simulink model "State_Flow_TestM"  (R2017a)
settings: Solver=FixedStepDiscrete  StartTime=0.0  StopTime=inf  FixedStep=0.001  RelTol=1e-3  EnableMultiTasking=on
values from neighbouring files (symbols this model uses):
  C = B    [testMatricePiccola.m]
libraries: xpcethercatlib x33, simulink x17, powerlib_meascontrol x3, commutil2 x2
(part 2 of 4)

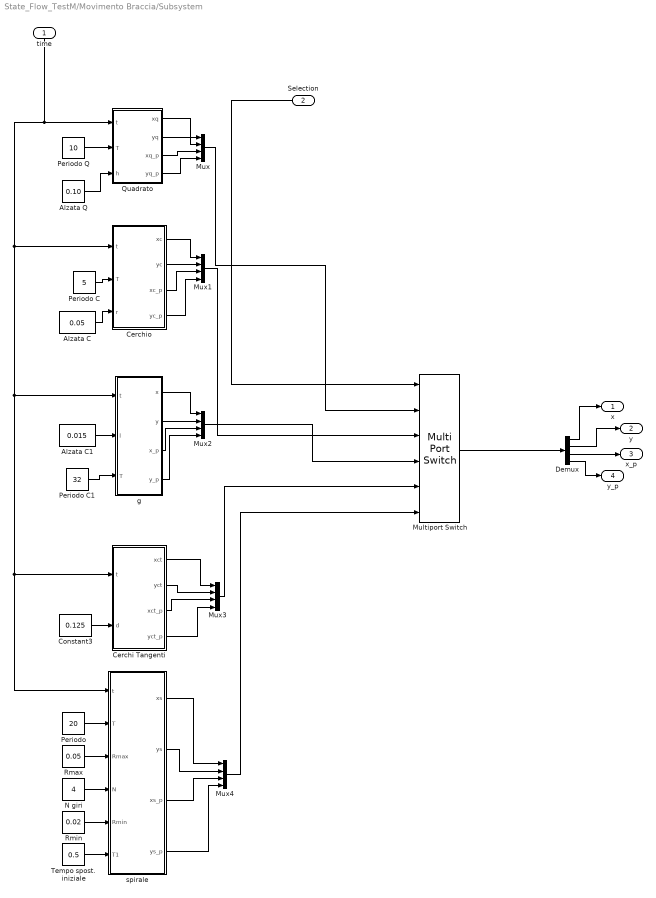
== system State_Flow_TestM/Movimento Braccia/Subsystem ==
  time : Inport
  Selection : Inport  Port=2
  Alzata C : Constant  Value=0.05
  Alzata C1 : Constant  Value=0.015
  Alzata Q : Constant  Value=0.10
  Cerchi Tangenti : MATLAB Function  TreatAsAtomicUnit=on
  Cerchio : MATLAB Function  TreatAsAtomicUnit=on
  Constant3 : Constant  Value=0.125
  Demux : Demux
  Multiport Switch : MultiPortSwitch  Inputs=5
  Mux{,1..4} (5 alike) : Mux
  N giri : Constant  Value=4
  Periodo : Constant  Value=20
  Periodo C : Constant  Value=5
  Periodo C1 : Constant  Value=32
  Periodo Q : Constant  Value=10
  Quadrato : MATLAB Function  TreatAsAtomicUnit=on
  Rmax : Constant  Value=0.05
  Rmin : Constant  Value=0.02
  Tempo spost. iniziale : Constant  Value=0.5
  g : MATLAB Function  TreatAsAtomicUnit=on
  spirale : MATLAB Function  TreatAsAtomicUnit=on
  x : Outport
  y : Outport  Port=2
  x_p : Outport  Port=3
  y_p : Outport  Port=4
  wires:
  Cerchio/2(yc) -> Mux1/2
  Cerchio/3(xc_p) -> Mux1/3
  Cerchio/4(yc_p) -> Mux1/4
  Cerchio/1(xc) -> Mux1/1
  Mux4/1 -> Multiport Switch/6
  Mux2/1 -> Multiport Switch/4
  spirale/4(ys_p) -> Mux4/4
  Quadrato/2(yq) -> Mux/2
  Quadrato/3(xq_p) -> Mux/3
  Quadrato/4(yq_p) -> Mux/4
  g/1(x) -> Mux2/1
  Demux/2 -> y/1
  Demux/1 -> x/1
  Selection/1 -> Multiport Switch/1
  time/1 -> Quadrato/1(t), Cerchio/1(t), g/1(t), Cerchi Tangenti/1(t), spirale/1(t)
  spirale/3(xs_p) -> Mux4/3
  spirale/2(ys) -> Mux4/2
  g/3(x_p) -> Mux2/3
  g/4(y_p) -> Mux2/4
  Cerchi Tangenti/2(yct) -> Mux3/2
  Cerchi Tangenti/1(xct) -> Mux3/1
  Cerchi Tangenti/4(yct_p) -> Mux3/4
  Cerchi Tangenti/3(xct_p) -> Mux3/3
  Quadrato/1(xq) -> Mux/1
  g/2(y) -> Mux2/2
  spirale/1(xs) -> Mux4/1
  Periodo C/1 -> Cerchio/2(T)
  Periodo Q/1 -> Quadrato/2(T)
  Alzata C/1 -> Cerchio/3(r)
  Alzata Q/1 -> Quadrato/3(h)
  Periodo/1 -> spirale/2(T)
  Constant3/1 -> Cerchi Tangenti/2(d)
  N giri/1 -> spirale/4(N)
  Rmin/1 -> spirale/5(Rmin)
  Tempo spost. iniziale/1 -> spirale/6(T1)
  Alzata C1/1 -> g/2(l)
  Periodo C1/1 -> g/3(T)
  Rmax/1 -> spirale/3(Rmax)
  Multiport Switch/1 -> Demux/1
  Mux3/1 -> Multiport Switch/5
  Mux/1 -> Multiport Switch/2
  Mux1/1 -> Multiport Switch/3
  Demux/3 -> x_p/1
  Demux/4 -> y_p/1

== system State_Flow_TestM/Movimento Braccia/Velocita vite  ==
  EtherCAT PDO Receive14 : xpcethercatlib/EtherCAT PDO Receive  Priority=2  sig_name=AZ1.Transmit PDO 1.Axis A Actual motor velocity  sig_offset=48  sig_type=int32  type_size=32  sig_dim=1  device_id=0  sample_time=0.001000
      settings: SourceProductName=Simulink Real-Time  SourceProductBaseCode=XP
  EtherCAT PDO Receive15 : xpcethercatlib/EtherCAT PDO Receive  Priority=2  sig_name=AZ1.Transmit PDO 2.Axis B Actual motor velocity  sig_offset=136  sig_type=int32  type_size=32  sig_dim=1  device_id=0  sample_time=0.001000
      settings: SourceProductName=Simulink Real-Time  SourceProductBaseCode=XP
  Vel Asse A conv : MATLAB Function  TreatAsAtomicUnit=on
  Vel Asse B conv : MATLAB Function  TreatAsAtomicUnit=on
  Velocity A : DataTypeConversion
  Velocity B : DataTypeConversion
  Asse B : Outport
  Asse A : Outport  Port=2
  wires:
  EtherCAT PDO Receive15/1 -> Velocity B/1
  EtherCAT PDO Receive14/1 -> Velocity A/1
  Vel Asse A conv/1(vel_A_conv) -> Asse A/1
  Velocity B/1 -> Vel Asse B conv/1(p)
  Vel Asse B conv/1(vel_B_conv) -> Asse B/1
  Velocity A/1 -> Vel Asse A conv/1(vA)

== system State_Flow_TestM/Out Asse A Braccia/Fungo ==
  In1 : Inport
  Constant : Constant  Value=0
  Data Type Conversion14 : DataTypeConversion
  Display10 : Display
  EtherCAT PDO Receive9 : xpcethercatlib/EtherCAT PDO Receive  Priority=2  sig_name=Beckoff.Channel 1.Input  sig_offset=0  sig_type=boolean  type_size=1  sig_dim=1  device_id=0  sample_time=0.001000
      settings: SourceProductName=Simulink Real-Time  SourceProductBaseCode=XP
  MATLAB Function : MATLAB Function  TreatAsAtomicUnit=on
  Memory : Memory
  Switch1 : Switch  Criteria=u2 ~= 0  Threshold=2
  Out1 : Outport
  wires:
  EtherCAT PDO Receive9/1 -> Data Type Conversion14/1
  Data Type Conversion14/1 -> MATLAB Function/2(old), Display10/1
  MATLAB Function/1(y) -> Memory/1
  In1/1 -> Switch1/3
  Memory/1 -> Switch1/2, MATLAB Function/1(now)
  Constant/1 -> Switch1/1
  Switch1/1 -> Out1/1

== system State_Flow_TestM/Out Asse B Braccia/Fungo ==
  In1 : Inport
  Constant : Constant  Value=0
  Data Type Conversion14 : DataTypeConversion
  Display10 : Display
  EtherCAT PDO Receive9 : xpcethercatlib/EtherCAT PDO Receive  Priority=2  sig_name=Beckoff.Channel 1.Input  sig_offset=0  sig_type=boolean  type_size=1  sig_dim=1  device_id=0  sample_time=0.001000
      settings: SourceProductName=Simulink Real-Time  SourceProductBaseCode=XP
  MATLAB Function : MATLAB Function  TreatAsAtomicUnit=on
  Memory : Memory
  Switch1 : Switch  Criteria=u2 ~= 0  Threshold=2
  Out1 : Outport
  wires:
  EtherCAT PDO Receive9/1 -> Data Type Conversion14/1
  Data Type Conversion14/1 -> MATLAB Function/2(old), Display10/1
  MATLAB Function/1(y) -> Memory/1
  In1/1 -> Switch1/3
  Memory/1 -> Switch1/2, MATLAB Function/1(now)
  Constant/1 -> Switch1/1
  Switch1/1 -> Out1/1

== system State_Flow_TestM/Out asse A Vite/Fungo ==
  In1 : Inport
  Constant : Constant  Value=0
  Data Type Conversion14 : DataTypeConversion
  Display10 : Display
  EtherCAT PDO Receive9 : xpcethercatlib/EtherCAT PDO Receive  Priority=2  sig_name=Beckoff.Channel 1.Input  sig_offset=0  sig_type=boolean  type_size=1  sig_dim=1  device_id=0  sample_time=0.001000
      settings: SourceProductName=Simulink Real-Time  SourceProductBaseCode=XP
  MATLAB Function : MATLAB Function  TreatAsAtomicUnit=on
  Memory : Memory
  Switch1 : Switch  Criteria=u2 ~= 0  Threshold=2
  Out1 : Outport
  wires:
  EtherCAT PDO Receive9/1 -> Data Type Conversion14/1
  Data Type Conversion14/1 -> MATLAB Function/2(old), Display10/1
  MATLAB Function/1(y) -> Memory/1
  In1/1 -> Switch1/3
  Memory/1 -> Switch1/2, MATLAB Function/1(now)
  Constant/1 -> Switch1/1
  Switch1/1 -> Out1/1

== system State_Flow_TestM/Out asse B Vite/Fungo ==
  In1 : Inport
  Constant : Constant  Value=0
  Data Type Conversion14 : DataTypeConversion
  Display10 : Display
  EtherCAT PDO Receive9 : xpcethercatlib/EtherCAT PDO Receive  Priority=2  sig_name=Beckoff.Channel 1.Input  sig_offset=0  sig_type=boolean  type_size=1  sig_dim=1  device_id=0  sample_time=0.001000
      settings: SourceProductName=Simulink Real-Time  SourceProductBaseCode=XP
  MATLAB Function : MATLAB Function  TreatAsAtomicUnit=on
  Memory : Memory
  Switch1 : Switch  Criteria=u2 ~= 0  Threshold=2
  Out1 : Outport
  wires:
  EtherCAT PDO Receive9/1 -> Data Type Conversion14/1
  Data Type Conversion14/1 -> MATLAB Function/2(old), Display10/1
  MATLAB Function/1(y) -> Memory/1
  In1/1 -> Switch1/3
  Memory/1 -> Switch1/2, MATLAB Function/1(now)
  Constant/1 -> Switch1/1
  Switch1/1 -> Out1/1

== system State_Flow_TestM/Sistema Braccia Linea/Velocita vite  ==
  EtherCAT PDO Receive14 : xpcethercatlib/EtherCAT PDO Receive  Priority=2  sig_name=AZ1.Transmit PDO 1.Axis A Actual motor velocity  sig_offset=48  sig_type=int32  type_size=32  sig_dim=1  device_id=0  sample_time=0.001000
      settings: SourceProductName=Simulink Real-Time  SourceProductBaseCode=XP
  EtherCAT PDO Receive15 : xpcethercatlib/EtherCAT PDO Receive  Priority=2  sig_name=AZ1.Transmit PDO 2.Axis B Actual motor velocity  sig_offset=136  sig_type=int32  type_size=32  sig_dim=1  device_id=0  sample_time=0.001000
      settings: SourceProductName=Simulink Real-Time  SourceProductBaseCode=XP
  Vel Asse A conv : MATLAB Function  TreatAsAtomicUnit=on
  Vel Asse B conv : MATLAB Function  TreatAsAtomicUnit=on
  Velocity A : DataTypeConversion
  Velocity B : DataTypeConversion
  Asse A : Outport
  Asse B : Outport  Port=2
  wires:
  EtherCAT PDO Receive15/1 -> Velocity B/1
  EtherCAT PDO Receive14/1 -> Velocity A/1
  Vel Asse A conv/1(vel_A_conv) -> Asse A/1
  Velocity B/1 -> Vel Asse B conv/1(p)
  Vel Asse B conv/1(vel_B_conv) -> Asse B/1
  Velocity A/1 -> Vel Asse A conv/1(vA)

== system State_Flow_TestM/Sistema Vite/Actual A ==
  Pos : Inport
  Offset : Inport  Port=2
  Rif asse B : Inport  Port=3
  Discrete Derivative A : simulink/Discrete/Discrete Derivative  gainval=1.0  ICPrevScaledInput=0.0  OutMin=[]  OutMax=[]  OutDataType=fixdt(1, 16)  OutScaling=2^-10  DoSatur=off
  Display31 : Display
  Posizione attuale Vite A : Subsystem
  Sum : Sum  Inputs=|-+
  A attuale : Outport
  wires:
  Offset/1 -> Sum/1
  Posizione attuale Vite A/1(A Att) -> A attuale/1, Discrete Derivative A/1
  Sum/1 -> Posizione attuale Vite A/1(Comp Vite A)
  Rif asse B/1 -> Posizione attuale Vite A/2("Comp Vite B ")
  Pos/1 -> Sum/2
  Discrete Derivative A/1 -> Display31/1

== system State_Flow_TestM/Sistema Vite/Clock reale ==
  cr : Inport
  offset : Inport  Port=2
  Sum2 : Sum  Inputs=-+|
  Ck : Outport
  wires:
  Sum2/1 -> Ck/1
  offset/1 -> Sum2/1
  cr/1 -> Sum2/2

== system State_Flow_TestM/Sistema Vite/Coppia VIte A finale ==
  Pos : Inport
  Vel : Inport  Port=2
  Gain : Gain  Gain=300*1000/0.36
  Gain6 : Gain  Gain=7.5*1000/0.36
  Sum9 : Sum  Inputs=|++
  Coppia : Outport
  wires:
  Pos/1 -> Gain/1
  Sum9/1 -> Coppia/1
  Gain6/1 -> Sum9/2
  Vel/1 -> Gain6/1
  Gain/1 -> Sum9/1

== system State_Flow_TestM/Sistema Vite/Velocita vite  ==
  EtherCAT PDO Receive14 : xpcethercatlib/EtherCAT PDO Receive  Priority=2  sig_name=AZ2.Transmit PDO 1.Axis A Actual motor velocity  sig_offset=304  sig_type=int32  type_size=32  sig_dim=1  device_id=0  sample_time=0.001000
      settings: SourceProductName=Simulink Real-Time  SourceProductBaseCode=XP
  EtherCAT PDO Receive15 : xpcethercatlib/EtherCAT PDO Receive  Priority=2  sig_name=AZ2.Transmit PDO 2.Axis B Actual motor velocity  sig_offset=392  sig_type=int32  type_size=32  sig_dim=1  device_id=0  sample_time=0.001000
      settings: SourceProductName=Simulink Real-Time  SourceProductBaseCode=XP
  Vel Asse A conv : MATLAB Function  TreatAsAtomicUnit=on
  Vel Asse B conv : MATLAB Function  TreatAsAtomicUnit=on
  Velocity A : DataTypeConversion
  Velocity B : DataTypeConversion
  Asse A : Outport
  Asse B : Outport  Port=2
  wires:
  EtherCAT PDO Receive15/1 -> Velocity B/1
  EtherCAT PDO Receive14/1 -> Velocity A/1
  Vel Asse A conv/1(vel_A_conv) -> Asse A/1
  Velocity B/1 -> Vel Asse B conv/1(p), Vel Asse A conv/2(vB)
  Vel Asse B conv/1(vel_B_conv) -> Asse B/1
  Velocity A/1 -> Vel Asse A conv/1(vA)

== system State_Flow_TestM/State flow robot/Mov1/Clock reale ==
  cr : Inport
  offset : Inport  Port=2
  Sum2 : Sum  Inputs=-+|
  Ck : Outport
  wires:
  Sum2/1 -> Ck/1
  offset/1 -> Sum2/1
  cr/1 -> Sum2/2

== system State_Flow_TestM/Sistema Vite/Actual A/Posizione attuale Vite A ==
  Comp Vite A : Inport
  "Comp Vite B " : Inport  Port=2
  Asse A conv : MATLAB Function  TreatAsAtomicUnit=on
  Asse B conv v : MATLAB Function  TreatAsAtomicUnit=on
  Sum5 : Sum
  A Att : Outport
  wires:
  Asse A conv/1(pos_A_conv) -> Sum5/1
  Asse B conv v/1(pos_B_conv_v) -> Sum5/2
  Comp Vite A/1 -> Asse A conv/1(p)
  Sum5/1 -> A Att/1
  "Comp Vite B "/1 -> Asse B conv v/1(p)

== matlab function State_Flow_TestM/Movimento Braccia/Cinematica Inversa1 ==
  data: x0old input; y0old input; theta1_0 input; theta2_0 input; time input; x0 output; y0 output
function [x0, y0] = fcn(x0old, y0old, theta1_0, theta2_0, time)

if time == 0 

d = 0.09; 
l = 0.25;

A = l^2*(sin(theta2_0)-sin(theta1_0))^2 + (-2*d -l*(cos(theta2_0)-cos(theta1_0)))^2;
B = -2*l^2*d*(sin(theta2_0)-sin(theta1_0))*(cos(theta2_0)+cos(theta1_0)) + ...
    l*(sin(theta2_0)-sin(theta1_0))*(-2*d -l*(cos(theta2_0)-cos(theta1_0)))*(-2*d -2*l*cos(theta2_0)) - ...
    2*l*sin(theta2_0)*(-2*d -l*(cos(theta2_0)-cos(theta1_0)))^2;
C = l^2*d^2*(cos(theta2_0)+cos(theta1_0))^2 -l*d*(cos(theta2_0)+cos(theta1_0))*(-2*d -l*(cos(theta2_0)-cos(theta1_0)))*(-2*d -2*l*cos(theta2_0)) + ...
    (d^2 + 2*d*l*cos(theta2_0))*(-2*d - l*(cos(theta2_0)-cos(theta1_0)))^2;

% Posizione Y end-effector
y0 = (-B + sqrt(B^2 - 4*A*C))/(2*A);
% Posizione X end-effector
x0 = (y0*l*(sin(theta2_0)-sin(theta1_0)) - l*d*(cos(theta2_0)+cos(theta1_0)))/(-2*d -l*(cos(theta2_0)-cos(theta1_0)));
else 
    x0 = x0old;
    y0 = y0old;
end

== matlab function State_Flow_TestM/Movimento Braccia/MATLAB Function ==
  data: x input; xp output; y input; yp output; bool input
function [xp,yp] = fcn(x, y, bool)
if bool == 4
    xp = x;
    yp = y;
else
    xp = 0;
    yp = 0;
end

== matlab function State_Flow_TestM/Sistema Braccia Linea/Velocita vite /Vel Asse A conv ==
  data: vA input; vel_A_conv output
function vel_A_conv = fcn(vA)
vel_A_conv = (vA)  *(2*pi)/163840/64;

== matlab function State_Flow_TestM/Sistema Braccia Linea/Velocita vite /Vel Asse B conv ==
  data: p input; vel_B_conv output
function vel_B_conv = fcn(p)
vel_B_conv = p  *(2*pi)/163840/64;

== matlab function State_Flow_TestM/Sistema Vite/Actual A/Posizione attuale Vite A/Asse A conv ==
  data: p input; pos_A_conv output
function pos_A_conv = fcn(p)
pos_A_conv = p * 0.02/(2*pi) * pi/2048/40;

== matlab function State_Flow_TestM/Sistema Vite/Rifermento Asse A Vite ==
  data: t input; ldm_pos output; h input; T input; ldm_vel output
function [ldm_pos, ldm_vel] = fcn(t,h,T)

xv = 0.3;
 x = t/T;
Ca=1/(xv*(1-xv));
Cv = 1/(1-xv);

if( x>= 0 && x < xv)
    f = Ca;
    F = Ca*x;
    G= Ca*x^2/2;
elseif(x >= xv && x < (1-xv) )
    f = 0;
    F = Cv;
    G= Ca*xv^2/2 + Cv*(x-xv);
elseif( x >= (1-xv) && x <= 1 )
    f = -Ca;
    xloc = x-(1-xv);
    F = Cv -Ca*xloc;
    G= Ca*xv^2/2 + Cv*(1-2*xv) + Cv*xloc -Ca*xloc^2/2;
else
    f=0;
    F=0;
    G= Ca*xv^2/2 + Cv*(1-2*xv) + Cv*xv -Ca*xv^2/2;
end

ldm_pos = G*h;
ldm_vel = F*h/T;

== matlab function State_Flow_TestM/LED Status/MATLAB Function ==
  data: u input; y output
function y = fcn(u)
if u == 2 ||u == 3
    y = 1;
else
    y = 0;
end

== matlab function State_Flow_TestM/LED Status/MATLAB Function1 ==
  data: u input; y output
function y = fcn(u)
if u == 1 || u == 2 || u == 4
    y = 1;
else
    y = 0;
end

== matlab function State_Flow_TestM/LED Status/MATLAB Function2 ==
  data: u input; y output
function y = fcn(u)
if u == 4 || u == 5
    y = 1;
else
    y = 0;
end

== matlab function State_Flow_TestM/Sistema Vite/Asse B conv ==
  data: p input; pos_B_conv output
function pos_B_conv = fcn(p)
pos_B_conv = p * pi/2048/40;

== matlab function State_Flow_TestM/Sistema Vite/Asse B ==
  data: t input; ldm_pos output; h input; T input; ldm_vel output
function [ldm_pos, ldm_vel] = fcn(t,h,T)

xv = 0.3;
 x = t/T;
Ca=1/(xv*(1-xv));
Cv = 1/(1-xv);

if( x>= 0 && x < xv)
    f = Ca;
    F = Ca*x;
    G= Ca*x^2/2;
elseif(x >= xv && x < (1-xv) )
    f = 0;
    F = Cv;
    G= Ca*xv^2/2 + Cv*(x-xv);
elseif( x >= (1-xv) && x <= 1 )
    f = -Ca;
    xloc = x-(1-xv);
    F = Cv -Ca*xloc;
    G= Ca*xv^2/2 + Cv*(1-2*xv) + Cv*xloc -Ca*xloc^2/2;
else
    f=0;
    F=0;
    G= Ca*xv^2/2 + Cv*(1-2*xv) + Cv*xv -Ca*xv^2/2;
end

ldm_pos = G*h;
ldm_vel = F*h/T;

== matlab function State_Flow_TestM/Sistema Vite/Actual A/Posizione attuale Vite A/Asse B conv v ==
  data: p input; pos_B_conv_v output
function pos_B_conv_v = fcn(p)
pos_B_conv_v = p * 0.02/(2*pi) * pi/2048/40;

== matlab function State_Flow_TestM/Sistema Vite/Velocita vite /Vel Asse A conv ==
  data: vA input; vel_A_conv output; vB input
function vel_A_conv = fcn(vA, vB)
vel_A_conv = (vA+vB) * 0.02/(2*pi) * pi/20480/40;

== matlab function State_Flow_TestM/Sistema Vite/Velocita vite /Vel Asse B conv ==
  data: p input; vel_B_conv output
function vel_B_conv = fcn(p)
vel_B_conv = p  * pi/20480/40;

== stateflow chart State_Flow_TestM/State flow robot ==
  settings: sampleTime=0.001
  state Step1
    entry:
    Bool = -1;
  state Step2
    entry:
    CoppiaH = 0;
  state SetA
    entry:
    CoppiaA = 0;
    C1 = 0;
  state OffSet
    entry:
    CoppiaH = 0;
    CoppiaA = 0;
    CoppiaB = 0;
    OffA = posA;
    OffB = posB;
    OffA_0 = posA;
    OffB_0 = posB;
    Bool = 2;
    Luci = 3;
    Hv = 1;
  state SetB1
    entry:
    CoppiaB = 0;
    C2 = 0;
  state Discesa_Vite
    entry:
    OffA_vite = posA_vite;
    CoppiaH=700;
  state Traiettoria
    entry:
    OffT = Clock;
    OffA_vite = posA_vite;
    OffB_vite = posB_vite;
    Luci = 4;
    Bool = 4;
    Hb = 1;
  state Step4
    entry:
    Bool = 0;
    Enable = 1;
  state Test_Kp
    entry:
    Bool = 5;
    Luci = 5;
    Kp = Kp + 500;
  state Controllo
    entry:
    Bool = 5;
    Luci = 5;
  state Coppie
    entry:
    OffA_0 = posA;
    OffB_0 = posB;
    CoppiaA = 250;
    CoppiaB = 250;
    CoppiaH = 0;
    Luci = 2;
  state SetB
    entry:
    CoppiaB = 0;
    C2 = 0;
  state SetA1
    entry:
    CoppiaA = 0;
    C1 = 0;
  state Home
    entry:
    [CoppiaA, CoppiaB, CoppiaH] = Homing(fc, fcA, fcB);
    Bool = 1;
    conv =  (2*pi)/16384/64;
    conv_vite = 0.02/(2*pi) * pi/2048/40;
    Luci = 1;
    C1 = 1;
    C2 = 1;
    Kp = KP;
    Hb = 0;
    Hv = 0;
  state Step3
    entry:
    CoppiaA = 0;
    CoppiaB = 0;
  state [CA,CB,CH] = Homing(fc,fcA,fcB) [function]
  state [CA,CB] = Mov1(posA,OffA,posB,OffB,OffT,Clock) [function] [commented out]
  state [CA,CB] = Mov(posA,OffA,posB,OffB,Clock, OffT, velA, velB) [function] [commented out]
  (default) -> Step1
  Step1 -> Step4 : [Status==1079 && avvio == 1]
  Home -> Step2 [order 2] : [fc==0]
  Coppie -> SetA [order 1] : [posA - OffA_0 >= 110*pi/180/conv]
  Step2 -> Coppie : [fcA == 1 && fcB==1]
  Discesa_Vite -> OffSet [order 1] : [posA_vite - OffA_vite >= 0.038/conv_vite]
  SetA -> SetB1 : [posB - OffB_0 >= 40*pi/180/conv]
  SetB1 -> Discesa_Vite : [C2 == 0]
  Traiettoria -> Test_Kp : after(6,sec)
  Test_Kp -> Controllo [order 2] : [Kp >= 7000]
  OffSet -> Traiettoria : [BeginWork == 1]
  Step4 -> Home : [HomeSignal == 1]
  Test_Kp -> OffSet [order 1] : [Kp < 7000]
  SetA1 -> Discesa_Vite : [C1 == 0]
  Discesa_Vite -> ? [order 1]
  SetB -> SetA1 : [posA - OffA_0 >= 110*pi/180/conv]
  Coppie -> SetB [order 2] : [posB - OffB_0 >= 40*pi/180/conv]
  Step3 -> Coppie : [fc==0]
  Home -> Step3 [order 1] : [fcA==1 && fcB==1]
  data: fc function_input double size=1; CA function_output; CB function_output; CH function_output; fcA function_input double size=1; fcB function_input double size=1; posA function_input double size=1; CA function_output double size=1; CB function_output double size=1; OffA function_input double size=1; posB function_input double size=1; OffB function_input double size=1; OffT function_input double size=1; Clock function_input double size=1; CA function_output double size=1; CB function_output double size=1; posA function_input double size=1; OffA function_input double size=1; posB function_input double size=1; OffB function_input double size=1; Clock function_input double size=1; OffT function_input double size=1; velA function_input double size=1; velB function_input double size=1; Clock input; posA_vite input; posB_vite input; SampleTime constant double; Status input; fc input; posA input; posB input; Bool output; OffT output; CoppiaH output; OffA_vite output; OffB_vite output; OffA output; OffB output; CoppiaA output; CoppiaB output; fcA input; fcB input; conv local; Luci output; OffA_0 local; OffB_0 local; C1 local; C2 local; conv_vite local; Kp output; KP input; Hv output; Hb output; HomeSignal input; avvio input; BeginWork input; Enable output

== matlab function State_Flow_TestM/Movimento Braccia/Cinematica Inversa ==
  data: x input; theta1 output; y input; theta2 output
function [theta1, theta2] = fcn(x, y)

d = 0.09; 
l = 0.25;

p = 2*d*l + 2*x*l;
e = 2*y*l;
f = x^2 + d^2 + y^2 + 2*x*d;
a = -2*d*l + 2*x*l;
b = +2*y*l;
c = x^2 + d^2 + y^2 - 2*x*d;



   theta1 = 2*atan2(e + sqrt(p^2 + e^2 -f^2), p +f);


   theta2 = 2*atan2(b - sqrt(a^2 + b^2 -c^2), a +c);
   if (theta2) < -deg2rad(200)
       theta2 = theta2 + 2*pi;
   end

== matlab function State_Flow_TestM/Movimento Braccia/Asse B conv brac1 ==
  data: p input; pos_B_conv output
function pos_B_conv = fcn(p)
pos_B_conv = p * (2*pi)/16384/64;

== matlab function State_Flow_TestM/State flow robot/Homing/MATLAB Function ==
  data: fc input; CA output; fcA input; fcB input; CB output; CH output
function [CA, CB, CH] = fcn(fc, fcA, fcB)

CA = -250;
CB = -250;
CH = -600;

if fc < 1
    CH = 0;
end
if fcA == 1
    CA = 0;
end
if fcB == 1
    CB = 0;
end

== matlab function State_Flow_TestM/Out asse A Vite/Fungo/MATLAB Function ==
  data: now input; old input; y output
function y = fcn(now, old)
if old == 0 && now == 1
    y = 1;
else
    y = old;
end

== matlab function State_Flow_TestM/Out asse B Vite/Fungo/MATLAB Function ==
  data: now input; old input; y output
function y = fcn(now, old)
if old == 0 && now == 1
    y = 1;
else
    y = old;
end

== matlab function State_Flow_TestM/Out Asse A Braccia/Fungo/MATLAB Function ==
  data: now input; old input; y output
function y = fcn(now, old)
if old == 0 && now == 1
    y = 1;
else
    y = old;
end

== matlab function State_Flow_TestM/Out Asse B Braccia/Fungo/MATLAB Function ==
  data: now input; old input; y output
function y = fcn(now, old)
if old == 0 && now == 1
    y = 1;
else
    y = old;
end

== matlab function State_Flow_TestM/State flow robot/Mov/Cinematica Inversa ==
  data: x input; theta1 output; y input; theta2 output
function [theta1, theta2] = fcn(x, y)

d = 0.09; 
l = 0.25;

p = 2*d*l + 2*x*l;
e = 2*y*l;
f = x^2 + d^2 + y^2 + 2*x*d;
a = -2*d*l + 2*x*l;
b = +2*y*l;
c = x^2 + d^2 + y^2 - 2*x*d;



   theta1 = 2*atan2(e + sqrt(p^2 + e^2 -f^2), p +f);


   theta2 = 2*atan2(b - sqrt(a^2 + b^2 -c^2), a +c);
   if (theta2) < -deg2rad(200)
       theta2 = theta2 + 2*pi;
   end

== matlab function State_Flow_TestM/State flow robot/Mov/Cinematica Inversa vel ==
  data: theta1 input; theta2 input; x input; y input; xp input; theta1_p output; yp input; theta2_p output
function [theta1_p, theta2_p] = fcn(theta1, theta2,x, y, xp, yp)

d = 0.09; 
l = 0.25;

N21 = -l*sin(theta1)*(x+d-l*cos(theta1)) + l*cos(theta1)*(y-l*sin(theta1));

N22 = -l*cos(theta2)*(y-l*sin(theta2))*(x+d-l*cos(theta1))/(x-d-l*cos(theta2)) + l*sin(theta2)*(x+d-l*cos(theta1));

D2 = y-l*sin(theta1) - (y-l*sin(theta2))*(x+d-l*cos(theta1))/(x-d-l*cos(theta2));

J21 = N21/D2;

J22 = N22/D2;

J11 = -(y-l*sin(theta2))/(x-d-l*cos(theta2))*(J21);

J12 = -(y-l*sin(theta2))/(x-d-l*cos(theta2))*(J22) -l*sin(theta2) + (y-l*sin(theta2))/(x-d-l*cos(theta2))*(l*cos(theta2));

J = [J11 J12; J21 J22];

theta_p = J^-1 * [xp; yp];
theta1_p = theta_p(1);
theta2_p = theta_p(2);

== matlab function State_Flow_TestM/State flow robot/Mov1/Asse A conv bracc ==
  data: p input; pos_A_conv output
function pos_A_conv = fcn(p)
pos_A_conv = p * (2*pi)/16384/64;

== matlab function State_Flow_TestM/State flow robot/Mov1/Asse A conv bracc1 ==
  data: p input; pos_A_conv output
function pos_A_conv = fcn(p)
pos_A_conv = p * (2*pi)/16384/64;

== matlab function State_Flow_TestM/State flow robot/Mov1/Ldm theta1 ==
  data: t input; theta1 output; T1 input
function theta1 = fcn(t,T1)
theta1 = T1(t*1000);
end

== matlab function State_Flow_TestM/State flow robot/Mov1/Ldm theta2 ==
  data: t input; theta1 output; T1 input
function theta1 = fcn(t,T1)
theta1 = T1(t*1000);
end

== matlab function State_Flow_TestM/State flow robot/Mov/x ==
  data: t input; ldm_pos output; h input; T input; ldm_vel output
function [ldm_pos, ldm_vel] = fcn(t,h,T)

xv = 0.3;
 x = t/T;
Ca=1/(xv*(1-xv));
Cv = 1/(1-xv);

if( x>= 0 && x < xv)
    f = Ca;
    F = Ca*x;
    G= Ca*x^2/2;
elseif(x >= xv && x < (1-xv) )
    f = 0;
    F = Cv;
    G= Ca*xv^2/2 + Cv*(x-xv);
elseif( x >= (1-xv) && x <= 1 )
    f = -Ca;
    xloc = x-(1-xv);
    F = Cv -Ca*xloc;
    G= Ca*xv^2/2 + Cv*(1-2*xv) + Cv*xloc -Ca*xloc^2/2;
else
    f=0;
    F=0;
    G= Ca*xv^2/2 + Cv*(1-2*xv) + Cv*xv -Ca*xv^2/2;
end

ldm_pos = G*h;
ldm_vel = F*h/T;

== matlab function State_Flow_TestM/State flow robot/Mov/Asse A conv bracc2 ==
  data: p input; pos_A_conv output
function pos_A_conv = fcn(p)
pos_A_conv = p * (2*pi)/16384/64;

== matlab function State_Flow_TestM/State flow robot/Mov/y ==
  data: t input; ldm_pos output; h input; T input; ldm_vel output
function [ldm_pos, ldm_vel] = fcn(t,h,T)

xv = 0.3;
 x = t/T;
Ca=1/(xv*(1-xv));
Cv = 1/(1-xv);

if( x>= 0 && x < xv)
    f = Ca;
    F = Ca*x;
    G= Ca*x^2/2;
elseif(x >= xv && x < (1-xv) )
    f = 0;
    F = Cv;
    G= Ca*xv^2/2 + Cv*(x-xv);
elseif( x >= (1-xv) && x <= 1 )
    f = -Ca;
    xloc = x-(1-xv);
    F = Cv -Ca*xloc;
    G= Ca*xv^2/2 + Cv*(1-2*xv) + Cv*xloc -Ca*xloc^2/2;
else
    f=0;
    F=0;
    G= Ca*xv^2/2 + Cv*(1-2*xv) + Cv*xv -Ca*xv^2/2;
end

ldm_pos = G*h;
ldm_vel = F*h/T;

== matlab function State_Flow_TestM/State flow robot/Mov/Asse B conv brac ==
  data: p input; pos_B_conv output
function pos_B_conv = fcn(p)
pos_B_conv = p * (2*pi)/16384/64;

== matlab function State_Flow_TestM/State flow robot/Mov/Cinematica Inversa1 ==
  data: theta1_0 input; x0 output; theta2_0 input; y0 output
function [x0, y0] = fcn(theta1_0, theta2_0)

d = 0.09; 
l = 0.25;

A = l^2*(sin(theta2_0)-sin(theta1_0))^2 + (-2*d -l*(cos(theta2_0)-cos(theta1_0)))^2;
B = -2*l^2*d*(sin(theta2_0)-sin(theta1_0))*(cos(theta2_0)+cos(theta1_0)) + ...
    l*(sin(theta2_0)-sin(theta1_0))*(-2*d -l*(cos(theta2_0)-cos(theta1_0)))*(-2*d -2*l*cos(theta2_0)) - ...
    2*l*sin(theta2_0)*(-2*d -l*(cos(theta2_0)-cos(theta1_0)))^2;
C = l^2*d^2*(cos(theta2_0)+cos(theta1_0))^2 -l*d*(cos(theta2_0)+cos(theta1_0))*(-2*d -l*(cos(theta2_0)-cos(theta1_0)))*(-2*d -2*l*cos(theta2_0)) + ...
    (d^2 + 2*d*l*cos(theta2_0))*(-2*d - l*(cos(theta2_0)-cos(theta1_0)))^2;

% Posizione Y end-effector
y0 = (-B + sqrt(B^2 - 4*A*C))/(2*A)
% Posizione X end-effector
x0 = (y0*l*(sin(theta2_0)-sin(theta1_0)) - l*d*(cos(theta2_0)+cos(theta1_0)))/(-2*d -l*(cos(theta2_0)-cos(theta1_0)))

== matlab function State_Flow_TestM/Sistema Braccia Linea/Asse A conv bracc2 ==
  data: p input; pos_A_conv output
function pos_A_conv = fcn(p)
pos_A_conv = p * (2*pi)/16384/64;

== matlab function State_Flow_TestM/Sistema Braccia Linea/Asse B conv brac1 ==
  data: p input; pos_B_conv output
function pos_B_conv = fcn(p)
pos_B_conv = p * (2*pi)/16384/64;

== matlab function State_Flow_TestM/Sistema Braccia Linea/Cinematica Inversa ==
  data: x input; theta1 output; y input; theta2 output
function [theta1, theta2] = fcn(x, y)

d = 0.09; 
l = 0.25;

p = 2*d*l + 2*x*l;
e = 2*y*l;
f = x^2 + d^2 + y^2 + 2*x*d;
a = -2*d*l + 2*x*l;
b = +2*y*l;
c = x^2 + d^2 + y^2 - 2*x*d;



   theta1 = 2*atan2(e + sqrt(p^2 + e^2 -f^2), p +f);


   theta2 = 2*atan2(b - sqrt(a^2 + b^2 -c^2), a +c);
   if (theta2) < -deg2rad(200)
       theta2 = theta2 + 2*pi;
   end

== matlab function State_Flow_TestM/Sistema Braccia Linea/Cinematica Inversa vel ==
  data: theta1 input; theta2 input; x input; y input; xp input; theta1_p output; yp input; theta2_p output
function [theta1_p, theta2_p] = fcn(theta1, theta2,x, y, xp, yp)

d = 0.09; 
l = 0.25;

N21 = -l*sin(theta1)*(x+d-l*cos(theta1)) + l*cos(theta1)*(y-l*sin(theta1));

N22 = -l*cos(theta2)*(y-l*sin(theta2))*(x+d-l*cos(theta1))/(x-d-l*cos(theta2)) + l*sin(theta2)*(x+d-l*cos(theta1));

D2 = y-l*sin(theta1) - (y-l*sin(theta2))*(x+d-l*cos(theta1))/(x-d-l*cos(theta2));

J21 = N21/D2;

J22 = N22/D2;

J11 = -(y-l*sin(theta2))/(x-d-l*cos(theta2))*(J21);

J12 = -(y-l*sin(theta2))/(x-d-l*cos(theta2))*(J22) -l*sin(theta2) + (y-l*sin(theta2))/(x-d-l*cos(theta2))*(l*cos(theta2));

J = [J11 J12; J21 J22];

theta_p = J^-1 * [xp; yp];
theta1_p = theta_p(1);
theta2_p = theta_p(2);

== matlab function State_Flow_TestM/Sistema Braccia Linea/Cinematica Inversa1 ==
  data: theta1_0 input; x0 output; theta2_0 input; y0 output
function [x0, y0] = fcn(theta1_0, theta2_0)

d = 0.09; 
l = 0.25;

A = l^2*(sin(theta2_0)-sin(theta1_0))^2 + (-2*d -l*(cos(theta2_0)-cos(theta1_0)))^2;
B = -2*l^2*d*(sin(theta2_0)-sin(theta1_0))*(cos(theta2_0)+cos(theta1_0)) + ...
    l*(sin(theta2_0)-sin(theta1_0))*(-2*d -l*(cos(theta2_0)-cos(theta1_0)))*(-2*d -2*l*cos(theta2_0)) - ...
    2*l*sin(theta2_0)*(-2*d -l*(cos(theta2_0)-cos(theta1_0)))^2;
C = l^2*d^2*(cos(theta2_0)+cos(theta1_0))^2 -l*d*(cos(theta2_0)+cos(theta1_0))*(-2*d -l*(cos(theta2_0)-cos(theta1_0)))*(-2*d -2*l*cos(theta2_0)) + ...
    (d^2 + 2*d*l*cos(theta2_0))*(-2*d - l*(cos(theta2_0)-cos(theta1_0)))^2;

% Posizione Y end-effector
y0 = (-B + sqrt(B^2 - 4*A*C))/(2*A)
% Posizione X end-effector
x0 = (y0*l*(sin(theta2_0)-sin(theta1_0)) - l*d*(cos(theta2_0)+cos(theta1_0)))/(-2*d -l*(cos(theta2_0)-cos(theta1_0)))

== matlab function State_Flow_TestM/Sistema Braccia Linea/x ==
  data: t input; ldm_pos output; h input; T input; ldm_vel output
function [ldm_pos, ldm_vel] = fcn(t,h,T)

xv = 0.3;
 x = t/T;
Ca=1/(xv*(1-xv));
Cv = 1/(1-xv);

if( x>= 0 && x < xv)
    f = Ca;
    F = Ca*x;
    G= Ca*x^2/2;
elseif(x >= xv && x < (1-xv) )
    f = 0;
    F = Cv;
    G= Ca*xv^2/2 + Cv*(x-xv);
elseif( x >= (1-xv) && x <= 1 )
    f = -Ca;
    xloc = x-(1-xv);
    F = Cv -Ca*xloc;
    G= Ca*xv^2/2 + Cv*(1-2*xv) + Cv*xloc -Ca*xloc^2/2;
else
    f=0;
    F=0;
    G= Ca*xv^2/2 + Cv*(1-2*xv) + Cv*xv -Ca*xv^2/2;
end

ldm_pos = G*h;
ldm_vel = F*h/T;

== matlab function State_Flow_TestM/Sistema Braccia Linea/y ==
  data: t input; ldm_pos output; h input; T input; ldm_vel output
function [ldm_pos, ldm_vel] = fcn(t,h,T)

xv = 0.3;
 x = t/T;
Ca=1/(xv*(1-xv));
Cv = 1/(1-xv);

if( x>= 0 && x < xv)
    f = Ca;
    F = Ca*x;
    G= Ca*x^2/2;
elseif(x >= xv && x < (1-xv) )
    f = 0;
    F = Cv;
    G= Ca*xv^2/2 + Cv*(x-xv);
elseif( x >= (1-xv) && x <= 1 )
    f = -Ca;
    xloc = x-(1-xv);
    F = Cv -Ca*xloc;
    G= Ca*xv^2/2 + Cv*(1-2*xv) + Cv*xloc -Ca*xloc^2/2;
else
    f=0;
    F=0;
    G= 1;
end

ldm_pos = G*h;
ldm_vel = F*h/T;

== matlab function State_Flow_TestM/Movimento Braccia/Asse A conv brac ==
  data: p input; pos_A_conv output
function pos_A_conv = fcn(p)
pos_A_conv = p * (2*pi)/16384/64;

== matlab function State_Flow_TestM/Movimento Braccia/Subsystem/Cerchio ==
  data: xc output; t input; yc output; T input; r input; xc_p output; yc_p output
function [xc, yc, xc_p, yc_p] = fcn(t, T, r)
xv = 0.4;
xj = 0.1;
x = t/T;
Ca = 1/((1-xv)*(xv-xj));
if ( x >= 0 && x < xj)            %acc crescente positiva
    f = Ca/xj*x;
    F = (1/2)*Ca/xj*x^2;
    G = (1/6)*Ca/xj*x^3;
    J = Ca/xj;

  elseif (x >= xj && x < (xv-xj))   %acc costante positiva
    f = Ca;
    F = Ca*x - (1/2)*Ca*xj;
    G = (1/2)*Ca*x^2 - (1/2)*Ca*xj*x + (1/6)*Ca*xj^2;
    J = 0;

  elseif( x>= (xv-xj) && x < xv)    %acc decrescente positiva
    f = -Ca/xj*x + Ca*xv/xj;
    F = -(1/2)*Ca/xj*x^2 + Ca/xj*xv*x - Ca*(xj + (1/2)/xj*xv^2 - xv);
    G = -(1/6)*Ca/xj*x^3 + (1/2)*Ca/xj*xv*x^2 - Ca*(xj + (1/2)/xj*xv^2 - xv)*x ...
        - (1/2)*Ca*xv^2  + (1/6)*Ca/xj*xv^3 + (1/2)*Ca*xv*xj;
    J = -Ca/xj;

  elseif( x>= xv && x < (1-xv))     %acc costante nulla
    f = 0;
    F = Ca*(xv - xj);
    G = Ca*(xv - xj)*x - (1/2)*Ca*xv^2 + (1/2)*Ca*xv*xj;
    J = 0;
    
  elseif( x>= (1-xv) && x < (1-xv+xj))   %acc decrescente negativa
    f = -Ca/xj*x + Ca/xj*(1-xv);
    F = -(1/2)*Ca/xj*x^2 + Ca/xj*(1-xv)*x + Ca*(xv-xj) - (1/2)*Ca/xj*(1-xv)^2;
    G = -(1/6)*Ca/xj*x^3 + (1/2)*Ca/xj*(1-xv)*x^2 + Ca*(xv-xj)*x - (1/2)*Ca/xj*(1-xv)^2*x ...
        - (1/2)*Ca*xv^2 + (1/2)*Ca*xv*xj + (1/6)*Ca/xj*(1-xv)^3;
    J = -Ca/xj;
    
  elseif( x>= (1-xv+xj) && x < (1-xj))   %acc costante negativa
    f = -Ca; 
    F = -Ca*x + Ca - (1/2)*Ca*xj;
    G = -(1/2)*Ca*x^2 + Ca*x - (1/2)*Ca*xj*x + 1 - Ca*(-(1/2)*xj + (1/6)*xj^2 + (1/2));
    J = 0;
    
  elseif( x>= (1-xj) && x <= 1)          %acc crescente negativa
    f = Ca/xj*(x-1);
    F = (1/2)*Ca/xj*x^2 - Ca/xj*x +(1/2)*Ca/xj;
    G = (1/6)*Ca/xj*x^3 - (1/2)*Ca/xj*x^2 +(1/2)*Ca/xj*x + 1 - (1/6)*Ca/xj;
    J = Ca/xj;
    
  else                                   %acc costante nulla
    f = 0;
    F = 0;
    G = 1;
    J = 0;
end
  
 alfa = G*2*pi;
 alfa_p = F*2*pi/T;
 xc = r*cos(pi/2-alfa);
 yc = r*sin(pi/2-alfa) - r;
 xc_p = r*sin(pi/2-alfa)*alfa_p;
 yc_p = -r*cos(pi/2-alfa)*alfa_p;

== matlab function State_Flow_TestM/Movimento Braccia/Subsystem/Quadrato ==
  data: xq output; yq output; t input; T input; h input; xq_p output; yq_p output
function [xq, yq, xq_p, yq_p] = fcn(t, T, h)
xv = 0.4;
xj = 0.1;
x1 = t/(0.5*T/4);
x2 = (t-0.5*T/4)/(T/4);
x3 = (t-1.5*T/4)/(T/4);
x4 = (t-2.5*T/4)/(T/4);
x5 = (t-3.5*T/4)/(0.5*T/4);
Ca = 1/((1-xv)*(xv-xj));
% Ca = 1/(xv*(1-xv));
% Cv = 1/(1-xv);


if t > 0 && t <= 0.5*T/4
  
  if ( x1 >= 0 && x1 < xj)            %acc crescente positiva
    f = Ca/xj*x1;
    F = (1/2)*Ca/xj*x1^2;
    G = (1/6)*Ca/xj*x1^3;
    J = Ca/xj;

  elseif (x1 >= xj && x1 < (xv-xj))   %acc costante positiva
    f = Ca;
    F = Ca*x1 - (1/2)*Ca*xj;
    G = (1/2)*Ca*x1^2 - (1/2)*Ca*xj*x1 + (1/6)*Ca*xj^2;
    J = 0;

  elseif( x1>= (xv-xj) && x1 < xv)    %acc decrescente positiva
    f = -Ca/xj*x1 + Ca*xv/xj;
    F = -(1/2)*Ca/xj*x1^2 + Ca/xj*xv*x1 - Ca*(xj + (1/2)/xj*xv^2 - xv);
    G = -(1/6)*Ca/xj*x1^3 + (1/2)*Ca/xj*xv*x1^2 - Ca*(xj + (1/2)/xj*xv^2 - xv)*x1 ...
        - (1/2)*Ca*xv^2  + (1/6)*Ca/xj*xv^3 + (1/2)*Ca*xv*xj;
    J = -Ca/xj;

  elseif( x1>= xv && x1 < (1-xv))     %acc costante nulla
    f = 0;
    F = Ca*(xv - xj);
    G = Ca*(xv - xj)*x1 - (1/2)*Ca*xv^2 + (1/2)*Ca*xv*xj;
    J = 0;
    
  elseif( x1>= (1-xv) && x1 < (1-xv+xj))   %acc decrescente negativa
    f = -Ca/xj*x1 + Ca/xj*(1-xv);
    F = -(1/2)*Ca/xj*x1^2 + Ca/xj*(1-xv)*x1 + Ca*(xv-xj) - (1/2)*Ca/xj*(1-xv)^2;
    G = -(1/6)*Ca/xj*x1^3 + (1/2)*Ca/xj*(1-xv)*x1^2 + Ca*(xv-xj)*x1 - (1/2)*Ca/xj*(1-xv)^2*x1 ...
        - (1/2)*Ca*xv^2 + (1/2)*Ca*xv*xj + (1/6)*Ca/xj*(1-xv)^3;
    J = -Ca/xj;
    
  elseif( x1>= (1-xv+xj) && x1 < (1-xj))   %acc costante negativa
    f = -Ca; 
    F = -Ca*x1 + Ca - (1/2)*Ca*xj;
    G = -(1/2)*Ca*x1^2 + Ca*x1 - (1/2)*Ca*xj*x1 + 1 - Ca*(-(1/2)*xj + (1/6)*xj^2 + (1/2));
    J = 0;
    
  elseif( x1>= (1-xj) && x1 <= 1)          %acc crescente negativa
    f = Ca/xj*(x1-1);
    F = (1/2)*Ca/xj*x1^2 - Ca/xj*x1 +(1/2)*Ca/xj;
    G = (1/6)*Ca/xj*x1^3 - (1/2)*Ca/xj*x1^2 +(1/2)*Ca/xj*x1 + 1 - (1/6)*Ca/xj;
    J = Ca/xj;
    
  else                                   %acc costante nulla
    f = 0;
    F = 0;
    G = 1;
    J = 0;
  end
    xq = G*h/2;
    xq_p = F*(h/2)/(T/4);
    yq = 0;
    yq_p = 0; 

elseif t > 0.5*T/4 && t <= 1.5*T/4
    Ca = 1/((1-xv)*(xv-xj));
% Cj = Ca/xj;
  
  if ( x2 >= 0 && x2 < xj)            %acc crescente positiva
    f = Ca/xj*x2;
    F = (1/2)*Ca/xj*x2^2;
    G = (1/6)*Ca/xj*x2^3;
    J = Ca/xj;

  elseif (x2 >= xj && x2 < (xv-xj))   %acc costante positiva
    f = Ca;
    F = Ca*x2 - (1/2)*Ca*xj;
    G = (1/2)*Ca*x2^2 - (1/2)*Ca*xj*x2 + (1/6)*Ca*xj^2;
    J = 0;

  elseif( x2>= (xv-xj) && x2 < xv)    %acc decrescente positiva
    f = -Ca/xj*x2 + Ca*xv/xj;
    F = -(1/2)*Ca/xj*x2^2 + Ca/xj*xv*x2 - Ca*(xj + (1/2)/xj*xv^2 - xv);
    G = -(1/6)*Ca/xj*x2^3 + (1/2)*Ca/xj*xv*x2^2 - Ca*(xj + (1/2)/xj*xv^2 - xv)*x2 ...
        - (1/2)*Ca*xv^2  + (1/6)*Ca/xj*xv^3 + (1/2)*Ca*xv*xj;
    J = -Ca/xj;

  elseif( x2>= xv && x2 < (1-xv))     %acc costante nulla
    f = 0;
    F = Ca*(xv - xj);
    G = Ca*(xv - xj)*x2 - (1/2)*Ca*xv^2 + (1/2)*Ca*xv*xj;
    J = 0;
    
  elseif( x2>= (1-xv) && x2 < (1-xv+xj))   %acc decrescente negativa
    f = -Ca/xj*x2 + Ca/xj*(1-xv);
    F = -(1/2)*Ca/xj*x2^2 + Ca/xj*(1-xv)*x2 + Ca*(xv-xj) - (1/2)*Ca/xj*(1-xv)^2;
    G = -(1/6)*Ca/xj*x2^3 + (1/2)*Ca/xj*(1-xv)*x2^2 + Ca*(xv-xj)*x2 - (1/2)*Ca/xj*(1-xv)^2*x2 ...
        - (1/2)*Ca*xv^2 + (1/2)*Ca*xv*xj + (1/6)*Ca/xj*(1-xv)^3;
    J = -Ca/xj;
    
  elseif( x2>= (1-xv+xj) && x2 < (1-xj))   %acc costante negativa
    f = -Ca; 
    F = -Ca*x2 + Ca - (1/2)*Ca*xj;
    G = -(1/2)*Ca*x2^2 + Ca*x2 - (1/2)*Ca*xj*x2 + 1 - Ca*(-(1/2)*xj + (1/6)*xj^2 + (1/2));
    J = 0;
    
  elseif( x2>= (1-xj) && x2 <= 1)          %acc crescente negativa
    f = Ca/xj*(x2-1);
    F = (1/2)*Ca/xj*x2^2 - Ca/xj*x2 +(1/2)*Ca/xj;
    G = (1/6)*Ca/xj*x2^3 - (1/2)*Ca/xj*x2^2 +(1/2)*Ca/xj*x2 + 1 - (1/6)*Ca/xj;
    J = Ca/xj;
    
  else                                   %acc costante nulla
    f = 0;
    F = 0;
    G = 1;
    J = 0;
  end
    xq = h/2;
    xq_p = 0;
    yq = -G*h; 
    yq_p = -F*h/(T/4); 

elseif t > 1.5*T/4 && t <= 2.5*T/4
     Ca = 1/((1-xv)*(xv-xj));
% Cj = Ca/xj;
  
  if ( x3 >= 0 && x3 < xj)            %acc crescente positiva
    f = Ca/xj*x3;
    F = (1/2)*Ca/xj*x3^2;
    G = (1/6)*Ca/xj*x3^3;
    J = Ca/xj;

  elseif (x3 >= xj && x3 < (xv-xj))   %acc costante positiva
    f = Ca;
    F = Ca*x3 - (1/2)*Ca*xj;
    G = (1/2)*Ca*x3^2 - (1/2)*Ca*xj*x3 + (1/6)*Ca*xj^2;
    J = 0;

  elseif( x3>= (xv-xj) && x3 < xv)    %acc decrescente positiva
    f = -Ca/xj*x3 + Ca*xv/xj;
    F = -(1/2)*Ca/xj*x3^2 + Ca/xj*xv*x3 - Ca*(xj + (1/2)/xj*xv^2 - xv);
    G = -(1/6)*Ca/xj*x3^3 + (1/2)*Ca/xj*xv*x3^2 - Ca*(xj + (1/2)/xj*xv^2 - xv)*x3 ...
        - (1/2)*Ca*xv^2  + (1/6)*Ca/xj*xv^3 + (1/2)*Ca*xv*xj;
    J = -Ca/xj;

  elseif( x3>= xv && x3 < (1-xv))     %acc costante nulla
    f = 0;
    F = Ca*(xv - xj);
    G = Ca*(xv - xj)*x3 - (1/2)*Ca*xv^2 + (1/2)*Ca*xv*xj;
    J = 0;
    
  elseif( x3>= (1-xv) && x3 < (1-xv+xj))   %acc decrescente negativa
    f = -Ca/xj*x3 + Ca/xj*(1-xv);
    F = -(1/2)*Ca/xj*x3^2 + Ca/xj*(1-xv)*x3 + Ca*(xv-xj) - (1/2)*Ca/xj*(1-xv)^2;
    G = -(1/6)*Ca/xj*x3^3 + (1/2)*Ca/xj*(1-xv)*x3^2 + Ca*(xv-xj)*x3 - (1/2)*Ca/xj*(1-xv)^2*x3 ...
        - (1/2)*Ca*xv^2 + (1/2)*Ca*xv*xj + (1/6)*Ca/xj*(1-xv)^3;
    J = -Ca/xj;
    
  elseif( x3>= (1-xv+xj) && x3 < (1-xj))   %acc costante negativa
    f = -Ca; 
    F = -Ca*x3 + Ca - (1/2)*Ca*xj;
    G = -(1/2)*Ca*x3^2 + Ca*x3 - (1/2)*Ca*xj*x3 + 1 - Ca*(-(1/2)*xj + (1/6)*xj^2 + (1/2));
    J = 0;
    
  elseif( x3>= (1-xj) && x3 <= 1)          %acc crescente negativa
    f = Ca/xj*(x3-1);
    F = (1/2)*Ca/xj*x3^2 - Ca/xj*x3 +(1/2)*Ca/xj;
    G = (1/6)*Ca/xj*x3^3 - (1/2)*Ca/xj*x3^2 +(1/2)*Ca/xj*x3 + 1 - (1/6)*Ca/xj;
    J = Ca/xj;
    
  else                                   %acc costante nulla
    f = 0;
    F = 0;
    G = 1;
    J = 0;
  end
    xq = h/2-G*h;
    xq_p = -F*h/(T/4);
    yq = -h; 
    yq_p = 0; 
 
elseif t > 2.5*T/4 && t <= 3.5*T/4
   Ca = 1/((1-xv)*(xv-xj));
% Cj = Ca/xj;
  
  if ( x4 >= 0 && x4 < xj)            %acc crescente positiva
    f = Ca/xj*x4;
    F = (1/2)*Ca/xj*x4^2;
    G = (1/6)*Ca/xj*x4^3;
    J = Ca/xj;

  elseif (x4 >= xj && x4 < (xv-xj))   %acc costante positiva
    f = Ca;
    F = Ca*x4 - (1/2)*Ca*xj;
    G = (1/2)*Ca*x4^2 - (1/2)*Ca*xj*x4 + (1/6)*Ca*xj^2;
    J = 0;

  elseif( x4>= (xv-xj) && x4 < xv)    %acc decrescente positiva
    f = -Ca/xj*x4 + Ca*xv/xj;
    F = -(1/2)*Ca/xj*x4^2 + Ca/xj*xv*x4 - Ca*(xj + (1/2)/xj*xv^2 - xv);
    G = -(1/6)*Ca/xj*x4^3 + (1/2)*Ca/xj*xv*x4^2 - Ca*(xj + (1/2)/xj*xv^2 - xv)*x4 ...
        - (1/2)*Ca*xv^2  + (1/6)*Ca/xj*xv^3 + (1/2)*Ca*xv*xj;
    J = -Ca/xj;

  elseif( x4>= xv && x4 < (1-xv))     %acc costante nulla
    f = 0;
    F = Ca*(xv - xj);
    G = Ca*(xv - xj)*x4 - (1/2)*Ca*xv^2 + (1/2)*Ca*xv*xj;
    J = 0;
    
  elseif( x4>= (1-xv) && x4 < (1-xv+xj))   %acc decrescente negativa
    f = -Ca/xj*x4 + Ca/xj*(1-xv);
    F = -(1/2)*Ca/xj*x4^2 + Ca/xj*(1-xv)*x4 + Ca*(xv-xj) - (1/2)*Ca/xj*(1-xv)^2;
    G = -(1/6)*Ca/xj*x4^3 + (1/2)*Ca/xj*(1-xv)*x4^2 + Ca*(xv-xj)*x4 - (1/2)*Ca/xj*(1-xv)^2*x4 ...
        - (1/2)*Ca*xv^2 + (1/2)*Ca*xv*xj + (1/6)*Ca/xj*(1-xv)^3;
    J = -Ca/xj;
    
  elseif( x4>= (1-xv+xj) && x4 < (1-xj))   %acc costante negativa
    f = -Ca; 
    F = -Ca*x4 + Ca - (1/2)*Ca*xj;
    G = -(1/2)*Ca*x4^2 + Ca*x4 - (1/2)*Ca*xj*x4 + 1 - Ca*(-(1/2)*xj + (1/6)*xj^2 + (1/2));
    J = 0;
    
  elseif( x4>= (1-xj) && x4 <= 1)          %acc crescente negativa
    f = Ca/xj*(x4-1);
    F = (1/2)*Ca/xj*x4^2 - Ca/xj*x4 +(1/2)*Ca/xj;
    G = (1/6)*Ca/xj*x4^3 - (1/2)*Ca/xj*x4^2 +(1/2)*Ca/xj*x4 + 1 - (1/6)*Ca/xj;
    J = Ca/xj;
    
  else                                   %acc costante nulla
    f = 0;
    F = 0;
    G = 1;
    J = 0;
  end
    xq = -h/2;
    xq_p = 0;
    yq = -h + G*h;
    yq_p = F*h/(T/4); 

elseif t > 3.5*T/4 && t <= 4*T/4
   Ca = 1/((1-xv)*(xv-xj));
% Cj = Ca/xj;
  
  if ( x5 >= 0 && x5 < xj)            %acc crescente positiva
    f = Ca/xj*x5;
    F = (1/2)*Ca/xj*x5^2;
    G = (1/6)*Ca/xj*x5^3;
    J = Ca/xj;

  elseif (x5 >= xj && x5 < (xv-xj))   %acc costante positiva
    f = Ca;
    F = Ca*x5 - (1/2)*Ca*xj;
    G = (1/2)*Ca*x5^2 - (1/2)*Ca*xj*x5 + (1/6)*Ca*xj^2;
    J = 0;

  elseif( x5>= (xv-xj) && x5 < xv)    %acc decrescente positiva
    f = -Ca/xj*x5 + Ca*xv/xj;
    F = -(1/2)*Ca/xj*x5^2 + Ca/xj*xv*x5 - Ca*(xj + (1/2)/xj*xv^2 - xv);
    G = -(1/6)*Ca/xj*x5^3 + (1/2)*Ca/xj*xv*x5^2 - Ca*(xj + (1/2)/xj*xv^2 - xv)*x5 ...
        - (1/2)*Ca*xv^2  + (1/6)*Ca/xj*xv^3 + (1/2)*Ca*xv*xj;
    J = -Ca/xj;

  elseif( x5>= xv && x5 < (1-xv))     %acc costante nulla
    f = 0;
    F = Ca*(xv - xj);
    G = Ca*(xv - xj)*x5 - (1/2)*Ca*xv^2 + (1/2)*Ca*xv*xj;
    J = 0;
    
  elseif( x5>= (1-xv) && x5 < (1-xv+xj))   %acc decrescente negativa
    f = -Ca/xj*x5 + Ca/xj*(1-xv);
    F = -(1/2)*Ca/xj*x5^2 + Ca/xj*(1-xv)*x5 + Ca*(xv-xj) - (1/2)*Ca/xj*(1-xv)^2;
    G = -(1/6)*Ca/xj*x5^3 + (1/2)*Ca/xj*(1-xv)*x5^2 + Ca*(xv-xj)*x5 - (1/2)*Ca/xj*(1-xv)^2*x5 ...
        - (1/2)*Ca*xv^2 + (1/2)*Ca*xv*xj + (1/6)*Ca/xj*(1-xv)^3;
    J = -Ca/xj;
    
  elseif( x5>= (1-xv+xj) && x5 < (1-xj))   %acc costante negativa
    f = -Ca; 
    F = -Ca*x5 + Ca - (1/2)*Ca*xj;
    G = -(1/2)*Ca*x5^2 + Ca*x5 - (1/2)*Ca*xj*x5 + 1 - Ca*(-(1/2)*xj + (1/6)*xj^2 + (1/2));
    J = 0;
    
  elseif( x5>= (1-xj) && x5 <= 1)          %acc crescente negativa
    f = Ca/xj*(x5-1);
    F = (1/2)*Ca/xj*x5^2 - Ca/xj*x5 +(1/2)*Ca/xj;
    G = (1/6)*Ca/xj*x5^3 - (1/2)*Ca/xj*x5^2 +(1/2)*Ca/xj*x5 + 1 - (1/6)*Ca/xj;
    J = Ca/xj;
    
  else                                   %acc costante nulla
    f = 0;
    F = 0;
    G = 1;
    J = 0;
  end
    xq = -h/2 + G*h/2;
    xq_p = F*h/2/(T/4);
    yq = 0
    yq_p = 0; 
else
xq = 0;
yq = 0;
xq_p = 0;
yq_p = 0; 
end

== matlab function State_Flow_TestM/Movimento Braccia/Quadrato1 ==
  data: x output; t input; y output; T input; h input
function [x, y] = fcn(t, T, h)
X1 = linspace(0, h, 1000*T/4);
X2 = linspace(h, 0, 1000*T/4);
Y1 = linspace(0, -h, 1000*T/4);
Y2 = linspace(-h, 0, 1000*T/4);

if t > 0 && t <= T/4
    y = 0;
    x = X1(t*1000);
elseif t > T/4 && t <= 2*T/4
    x = h;
    y = Y1((t-T/4)*1000);
elseif t > 2*T/4 && t <= 3*T/4
    y = -h;
    x = X2((t-2*T/4)*1000);
elseif t > 3*T/4 && t <= 4*T/4
    x = 0;
    y = Y2((t-3*T/4)*1000);
else
x = 0;
y = 0;
end

== matlab function State_Flow_TestM/Movimento Braccia/Cinematica Inversa vel ==
  data: theta1 input; theta2 input; x input; y input; xp input; theta1_p output; yp input; theta2_p output
function [theta1_p, theta2_p] = fcn(theta1, theta2,x, y, xp, yp)

d = 0.09; 
l = 0.25;

N21 = -l*sin(theta1)*(x+d-l*cos(theta1)) + l*cos(theta1)*(y-l*sin(theta1));

N22 = -l*cos(theta2)*(y-l*sin(theta2))*(x+d-l*cos(theta1))/(x-d-l*cos(theta2)) + l*sin(theta2)*(x+d-l*cos(theta1));

D2 = y-l*sin(theta1) - (y-l*sin(theta2))*(x+d-l*cos(theta1))/(x-d-l*cos(theta2));

J21 = N21/D2;

J22 = N22/D2;

J11 = -(y-l*sin(theta2))/(x-d-l*cos(theta2))*(J21);

J12 = -(y-l*sin(theta2))/(x-d-l*cos(theta2))*(J22) -l*sin(theta2) + (y-l*sin(theta2))/(x-d-l*cos(theta2))*(l*cos(theta2));

J = [J11 J12; J21 J22];

theta_p = J^-1 * [xp; yp];
theta1_p = theta_p(1);
theta2_p = theta_p(2);

== matlab function State_Flow_TestM/Movimento Braccia/Velocita vite /Vel Asse A conv ==
  data: vA input; vel_A_conv output
function vel_A_conv = fcn(vA)
vel_A_conv = (vA)  *(2*pi)/163840/64;

== matlab function State_Flow_TestM/Movimento Braccia/Velocita vite /Vel Asse B conv ==
  data: p input; vel_B_conv output
function vel_B_conv = fcn(p)
vel_B_conv = p  *(2*pi)/163840/64;

== matlab function State_Flow_TestM/Movimento/MATLAB Function ==
  data: x input; xp output; y input; yp output; bool input
function [xp,yp] = fcn(x, y, bool)
if bool == 4
    xp = x;
    yp = y;
else
    xp = 0;
    yp = 0;
end

== matlab function State_Flow_TestM/Out Asse A Braccia/MATLAB Function ==
  data: C input; Cout output
function Cout = fcn(C)
if C >= 800 && C <= 1000
Cout = 1200;
elseif C >= 1700 && C <= 2000
Cout = 1500;
elseif C <= -800 && C >= -1000
Cout = -1200;
elseif C <= -1700 && C >= -2000
Cout = -1500; 
else 
Cout = C;
end

== matlab function State_Flow_TestM/Out Asse B Braccia/MATLAB Function ==
  data: C input; Cout output
function Cout = fcn(C)
if C >= 800 && C <= 1000
Cout = 1200;
elseif C >= 1700 && C <= 2000
Cout = 1500;
elseif C <= -800 && C >= -1000
Cout = -1200;
elseif C <= -1700 && C >= -2000
Cout = -1500; 
else 
Cout = C;
end
